simulink model "pmsm_simulink_r13"  (Simulink 5.1)
settings: Solver=ode5  StartTime=0.0  StopTime=0.5  FixedStep=0.1e-3  RelTol=1e-3
settings Model: LastModifiedBy=user  LimitDataPoints=off  ProdHWDeviceType=Microprocessor

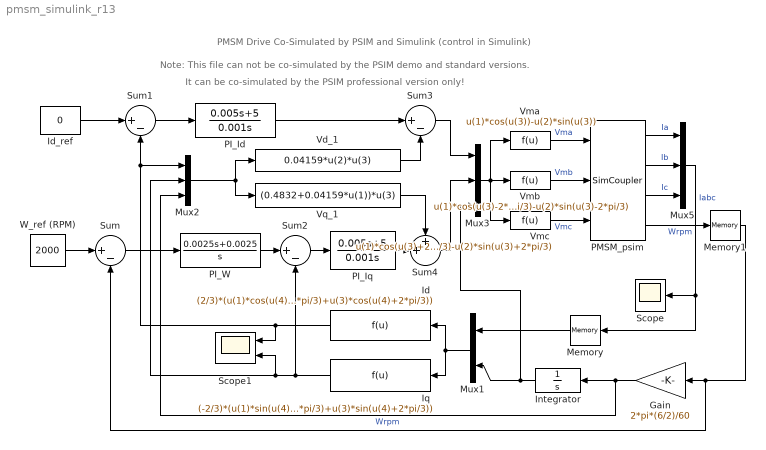
== system pmsm_simulink_r13 ==
  note: PMSM Drive Co-Simulated by PSIM and Simulink (control in Simulink)
  note: Note: This file can not be co-simulated by the PSIM demo and standard versions.
  note: It can be co-simulated by the PSIM professional version only!
  Gain : Gain  Orientation=left  Gain=2*pi*(6/2)/60  SaturateOnIntegerOverflow=on
  Id : Fcn  Orientation=left  Expr=(2/3)*(u(1)*cos(u(4))+u(2)*cos(u(4)-2*pi/3)+u(3)*cos(u(4)+2*pi/3))
  Id_ref : Constant  Value=0
  Integrator : Integrator  Orientation=left
  Iq : Fcn  Orientation=left  Expr=(-2/3)*(u(1)*sin(u(4))+u(2)*sin(u(4)-2*pi/3)+u(3)*sin(u(4)+2*pi/3))
  Memory : Memory  Orientation=left
  Memory1 : Memory
  Mux1 : Mux  Orientation=left  Inputs=2
  Mux2 : Mux  Inputs=3
  Mux3 : Mux  Inputs=3
  Mux5 : Mux  Inputs=3
  PI_Id : TransferFcn  Numerator=[0.005 5]  Denominator=[0.001 0]
  PI_Iq : TransferFcn  Numerator=[0.005 5]  Denominator=[0.001 0]
  PI_W : TransferFcn  Numerator=[0.0025 0.0025]  Denominator=[1 0]
  PMSM_psim : S-Function  FunctionName=SimCoupler  Parameters='C:\PSIM\examples\SimCoupler\PMSM_psim.sch'  mask(SimCoupler){Netlist_File=C:\PSIM6.1\examples\simcoupler\PMSM_psim.cct}
      mask prompts: Netlist_File "Model Netlist File"
      mask init:
      | c=[0:10:360]*pi/180;
      | x1=cos(c)*30; y1=sin(c)*30+20;
      | x2=cos(c)*30;y2=sin(c)*30-20;
      settings: OpenFcn=PSimDialog('PSimFileEdt','Value','Parameters');
      mask Display:
      | plot(-60,-60,60,60,x1,y1,x2,y2)
      | port_label('input', 1, 'Va')
      | port_label('input', 2, 'Vb')
      | port_label('input', 3, 'Vc')
      | port_label('output', 1, 'Ia')
      | port_label('output', 2, 'Ib')
      | port_label('output', 3, 'Ic')
      | port_label('output', 4, 'Wrpm')
  Scope : Scope
  Scope1 : Scope  NumInputPorts=2
      settings: TickLabels=on  TimeRange=0.5  YMin=-0.75~0  YMax=0.75~7.5  MaxDataPoints=500000
  Sum{,1..3} (4 alike) : Sum  Inputs=|+-  SaturateOnIntegerOverflow=on  InputSameDT=on
  Sum4 : Sum  Inputs=++|  SaturateOnIntegerOverflow=on  InputSameDT=on
  Vd_1 : Fcn  Expr=0.04159*u(2)*u(3)
  Vma : Fcn  Expr=u(1)*cos(u(3))-u(2)*sin(u(3))
  Vmb : Fcn  Expr=u(1)*cos(u(3)-2*pi/3)-u(2)*sin(u(3)-2*pi/3)
  Vmc : Fcn  Expr=u(1)*cos(u(3)+2*pi/3)-u(2)*sin(u(3)+2*pi/3)
  Vq_1 : Fcn  Expr=(0.4832+0.04159*u(1))*u(3)
  W_ref (RPM) : Constant  Value=2000
  wires:
  Gain/1 -> Integrator/1, Mux2/3  "Wrpm"
  Integrator/1 -> Mux1/2, Mux3/3
  Mux1/1 -> Id/1, Iq/1
  Id/1 -> Scope1/1, Sum1/2, Mux2/1
  Iq/1 -> Sum2/2, Mux2/2, Scope1/2
  W_ref (RPM)/1 -> Sum/1
  Id_ref/1 -> Sum1/1
  Sum1/1 -> PI_Id/1
  PI_Id/1 -> Sum3/1
  Sum/1 -> PI_W/1
  Sum2/1 -> PI_Iq/1
  Vd_1/1 -> Sum3/2
  PI_Iq/1 -> Sum4/2
  Vq_1/1 -> Sum4/1
  Mux2/1 -> Vd_1/1, Vq_1/1
  Sum3/1 -> Mux3/1
  Sum4/1 -> Mux3/2
  Mux3/1 -> Vma/1, Vmb/1, Vmc/1
  PI_W/1 -> Sum2/1
  Mux5/1 -> Scope/1, Memory/1  "Iabc"
  PMSM_psim/1 -> Mux5/1  "Ia"
  PMSM_psim/2 -> Mux5/2  "Ib"
  PMSM_psim/3 -> Mux5/3  "Ic"
  Vmb/1 -> PMSM_psim/2  "Vmb"
  Vmc/1 -> PMSM_psim/3  "Vmc"
  PMSM_psim/4 -> Memory1/1  "Wrpm"
  Vma/1 -> PMSM_psim/1  "Vma"
  Memory/1 -> Mux1/1
  Memory1/1 -> Gain/1, Sum/2
